simulink model "extra_blocks"  (R2023a)
settings: Solver=FixedStepDiscrete  StartTime=0.0  StopTime=inf  FixedStep=0.002  RelTol=1e-3  EnableMultiTasking=on
values from neighbouring files (symbols this model uses):
  a = 0    [simulate_hover.m]
  B = [0, 0, 0 ... (first row only)    [setup_lab_hover.m]    (also in simulate_hover.m = 0.042375883612; solveSyms3.m = evalin('base', 'B'))
  cycleGain = 0.2    [simulate_hover.m]    (also in temp.m = 1)
  Jp = 2*Jeq_prop    (= 0.0552224595625)    [setup_lab_hover.m]    (also in simulate_hover.m)
  Jr = 2*Jeq_prop    (= 0.0552224595625)    [setup_lab_hover.m]    (also in simulate_hover.m)
  Jy = 4*Jeq_prop    (= 0.110444919125)    [setup_lab_hover.m]    (also in simulate_hover.m)
  kd = 0.5    [simulate_hover.m]
  Kf = 0.1188    [setup_lab_hover.m]    (also in simulate_hover.m)
  Kt = 0.0036    [setup_lab_hover.m]    (also in simulate_hover.m)
  L = 7.75*0.0254    (= 0.19685)    [setup_lab_hover.m]    (also in simulate_hover.m = 0.1969)
  num1 = double(subs(u_1, {x1, x2, x3, x4, x5, x6, statey_der}, {v1, v2, v3, v4, v5, v6, v7}))    [solveSyms.m]
  num2 = double(subs(u_2, {x1, x2, x3, x4, x5, x6, u1}, {v1, v2, v3, v4, v5, v6, u1_num}))    [solveSyms.m]
  r = flexSize(no)    [phaseComp.m]    (also in simulate_hover.m = 0.5)
  skew = 2    [simulate_hover.m]
  u10_range = -199:100:401    [tempAdvanced.m]
  u1_range = -15:1:15    [tempAdvanced.m]
  V_bias = 12    [setup_lab_hover.m]    (also in simulate_hover.m)
  wcf = 2 * pi * 20    (= 125.663706144)    [setup_lab_hover.m]    (also in simulate_hover.m)
  x0 = x0(:)    [calc_jacob.m]    (also in setup_lab_hover.m = transpose(0.5*[pi/2, pi/6, pi/6, 0, 0, 0]))
  x5_range = -(29.5):10:(30.5)    [tempAdvanced.m]
  x6_range = -(29.5):10:(30.5)    [tempAdvanced.m]
  zetaf = 0.6    [setup_lab_hover.m]    (also in simulate_hover.m)
undefined symbols (not defined in the file or in its folder): Kp1_T, numBias, x1_range, x2_range
libraries: simulink_extras x3, quarc_library x2
settings Model: ExtModeTrigDuration=10000  Creator=kille  LastModifiedBy=Jacob
settings SolverCC: AlgebraicLoopSolver=TrustRegion  PositivePriorityOrder=on
settings DataIOCC: ReturnWorkspaceOutputs=off
settings OptimizationCC: LifeSpan=inf
settings DebuggingCC: UnconnectedInputMsg=warning  UnconnectedOutputMsg=warning  UnconnectedLineMsg=warning  ArithmeticOperatorsInVariantConditions=warning
settings ModelReferenceCC: EnableRefExpFcnMdlSchedulingChecks=on
settings SFSimCC: SimUseLocalCustomCode=off  CustomCodeUndefinedFunction=UseInterfaceOnly
settings RTWCC: Description=QUARC Win64 Target  SystemTargetFile=quarc_win64.tlc  TemplateMakefile=quarc_default_tmf  RTWUseLocalCustomCode=off
settings CodeAppCC: StateflowObjectComments=on
settings STFCustomTargetCC: TargetPreCompLibLocation=C:\PROGRA~3\QUARC\lib\2016a\win64\release  UseToolchainInfoCompliant=off  SystemTargetFile=quarc_win64.tlc
settings GRTTargetCC: TargetPreCompLibLocation=C:\PROGRA~3\QUARC\lib\2016a\win64\release  ParMdlRefBuildCompliant=off  CompOptLevelCompliant=off  CombineOutputUpdateFcns=off  MatFileLogging=off  CPPClassGenCompliant=off  GRTInterface=on  UseToolchainInfoCompliant=off  ExtMode=on  ExtModeMexFile=quarc_comm
settings ConfigComp: CovMetricSettings=dswe

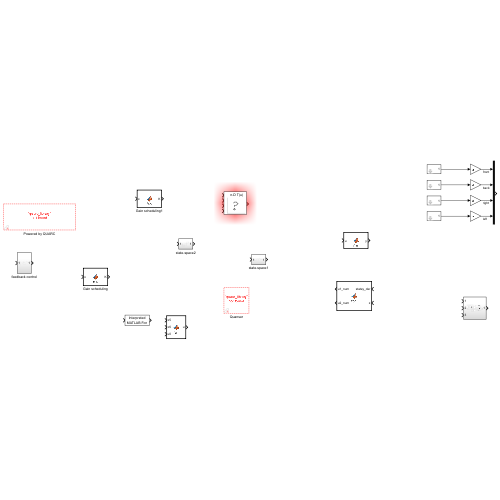
[thumbnail: Simulink's stored preview of the top-level diagram]
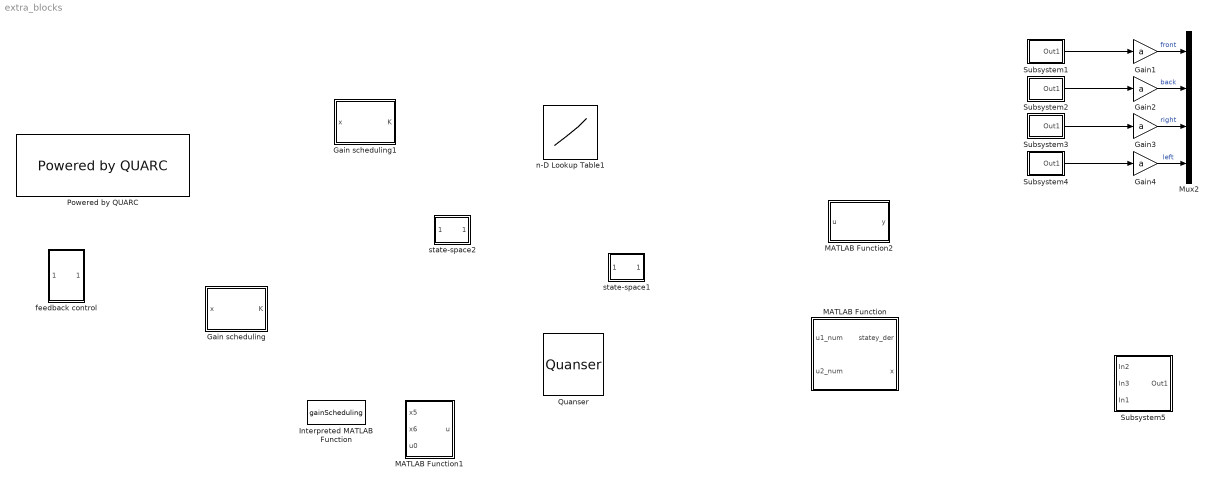
== system extra_blocks ==
  Gain scheduling : MATLAB Function  TreatAsAtomicUnit=on
  Gain scheduling1 : MATLAB Function  TreatAsAtomicUnit=on
  Gain{1..4} (4 alike) : Gain  Gain=a
  Interpreted MATLAB Function : MATLABFcn  MATLABFcn=gainScheduling  Output1D=off
  MATLAB Function : MATLAB Function  TreatAsAtomicUnit=on
  MATLAB Function1 : MATLAB Function  TreatAsAtomicUnit=on
  MATLAB Function2 : MATLAB Function  TreatAsAtomicUnit=on
  Mux2 : Mux
  Powered by QUARC : quarc_library/Logos/Powered by QUARC
  Quanser : quarc_library/Logos/Quanser
  Subsystem1 : Subsystem  mask{start_time=1, duration=1, amplitude=1}
      mask prompts: start_time "Start time"
  Subsystem2 : Subsystem  mask{start_time=6, duration=1, amplitude=1}
      mask prompts: start_time "Start time"
  Subsystem3 : Subsystem  mask{start_time=11, duration=1, amplitude=1}
      mask prompts: start_time "Start time"
  Subsystem4 : Subsystem  mask{start_time=16, duration=1, amplitude=1}
      mask prompts: start_time "Start time"
  Subsystem5 : Subsystem
  feedback control : Subsystem
  n-D Lookup Table1 : Lookup_n-D  NumberOfTableDimensions=4  BreakpointsForDimension1=x5_range  BreakpointsForDimension2=x6_range  BreakpointsForDimension3=u10_range  BreakpointsForDimension4=u20_range  Table=num2  InternalRulePriority=Speed  RndMeth=Simplest
      settings: InputPortMap=u0,u1,u2,u3
  state-space1 : Subsystem
  state-space2 : Subsystem
  wires:
  Subsystem2/1(Out1) -> Gain2/1
  Subsystem1/1(Out1) -> Gain1/1
  Subsystem3/1(Out1) -> Gain3/1
  Gain3/1 -> Mux2/3  "right"
  Gain4/1 -> Mux2/4  "left"
  Gain1/1 -> Mux2/1  "front"
  Gain2/1 -> Mux2/2  "back"
  Subsystem4/1(Out1) -> Gain4/1

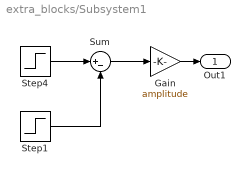
== system extra_blocks/Subsystem1 ==
  Gain : Gain  Gain=amplitude
  Step1 : Step  Time=start_time + duration  SampleTime=0
  Step4 : Step  Time=start_time  SampleTime=0
  Sum : Sum  Inputs=|+-
  Out1 : Outport
  wires:
  Gain/1 -> Out1/1
  Step1/1 -> Sum/2
  Step4/1 -> Sum/1
  Sum/1 -> Gain/1

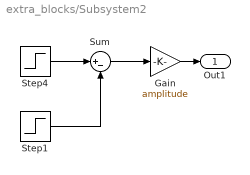
== system extra_blocks/Subsystem2 ==
  Gain : Gain  Gain=amplitude
  Step1 : Step  Time=start_time + duration  SampleTime=0
  Step4 : Step  Time=start_time  SampleTime=0
  Sum : Sum  Inputs=|+-
  Out1 : Outport
  wires:
  Gain/1 -> Out1/1
  Step1/1 -> Sum/2
  Step4/1 -> Sum/1
  Sum/1 -> Gain/1

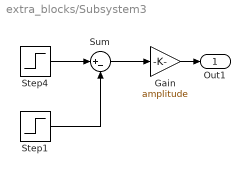
== system extra_blocks/Subsystem3 ==
  Gain : Gain  Gain=amplitude
  Step1 : Step  Time=start_time + duration  SampleTime=0
  Step4 : Step  Time=start_time  SampleTime=0
  Sum : Sum  Inputs=|+-
  Out1 : Outport
  wires:
  Gain/1 -> Out1/1
  Step1/1 -> Sum/2
  Step4/1 -> Sum/1
  Sum/1 -> Gain/1

== system extra_blocks/Subsystem4 ==
  Gain : Gain  Gain=amplitude
  Step1 : Step  Time=start_time + duration  SampleTime=0
  Step4 : Step  Time=start_time  SampleTime=0
  Sum : Sum  Inputs=|+-
  Out1 : Outport
  wires:
  Gain/1 -> Out1/1
  Step1/1 -> Sum/2
  Step4/1 -> Sum/1
  Sum/1 -> Gain/1

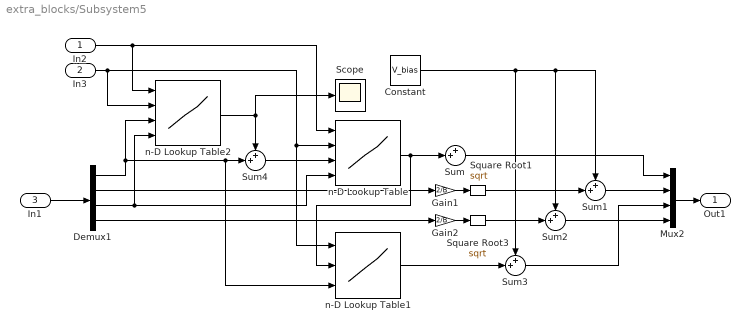
== system extra_blocks/Subsystem5 ==
  In2 : Inport
  In3 : Inport  Port=2
  In1 : Inport  Port=3
  Constant : Constant  Value=V_bias
  Demux1 : Demux
  Gain1 : Gain  Gain=2/B
  Gain2 : Gain  Gain=2/B
  Mux2 : Mux
  Scope : Scope
  Square Root1 : Sqrt
  Square Root3 : Sqrt
  Sum{,1..4} (5 alike) : Sum  Inputs=++|
  n-D Lookup Table : Lookup_n-D  NumberOfTableDimensions=4  BreakpointsForDimension1=x5_range  BreakpointsForDimension2=x6_range  BreakpointsForDimension3=u10_range  BreakpointsForDimension4=u20_range  Table=num1  InternalRulePriority=Speed  RndMeth=Simplest
      settings: InputPortMap=u0,u1,u2,u3
  n-D Lookup Table1 : Lookup_n-D  NumberOfTableDimensions=3  BreakpointsForDimension1=x6_range  BreakpointsForDimension2=u1_range  BreakpointsForDimension3=u10_range  BreakpointsForDimension4=u20_range  Table=num2  InternalRulePriority=Speed  RndMeth=Simplest
      settings: InputPortMap=u0,u1,u2
  n-D Lookup Table2 : Lookup_n-D  NumberOfTableDimensions=4  BreakpointsForDimension1=x5_range  BreakpointsForDimension2=x6_range  BreakpointsForDimension3=u10_range  BreakpointsForDimension4=u20_range  Table=numBias  InternalRulePriority=Speed  RndMeth=Simplest
      settings: InputPortMap=u0,u1,u2,u3
  Out1 : Outport
  wires:
  Demux1/2 -> Gain1/1
  In3/1 -> n-D Lookup Table2/2, n-D Lookup Table1/1, n-D Lookup Table/2
  n-D Lookup Table/1 -> Sum/2, n-D Lookup Table1/2
  Mux2/1 -> Out1/1
  Demux1/3 -> n-D Lookup Table2/4, n-D Lookup Table/4
  Gain2/1 -> Square Root3/1
  Demux1/4 -> Gain2/1
  In2/1 -> n-D Lookup Table2/1, n-D Lookup Table/1
  Gain1/1 -> Square Root1/1
  In1/1 -> Demux1/1
  Sum/1 -> Mux2/1
  Square Root3/1 -> Sum2/2
  Sum2/1 -> Mux2/4
  Square Root1/1 -> Sum1/2
  Sum1/1 -> Mux2/2
  Constant/1 -> Sum3/1, Sum2/1, Sum1/1
  Demux1/1 -> n-D Lookup Table1/3, Sum4/2, n-D Lookup Table2/3
  n-D Lookup Table2/1 -> Scope/1, Sum4/1
  n-D Lookup Table1/1 -> Sum3/2
  Sum3/1 -> Mux2/3
  Sum4/1 -> n-D Lookup Table/3

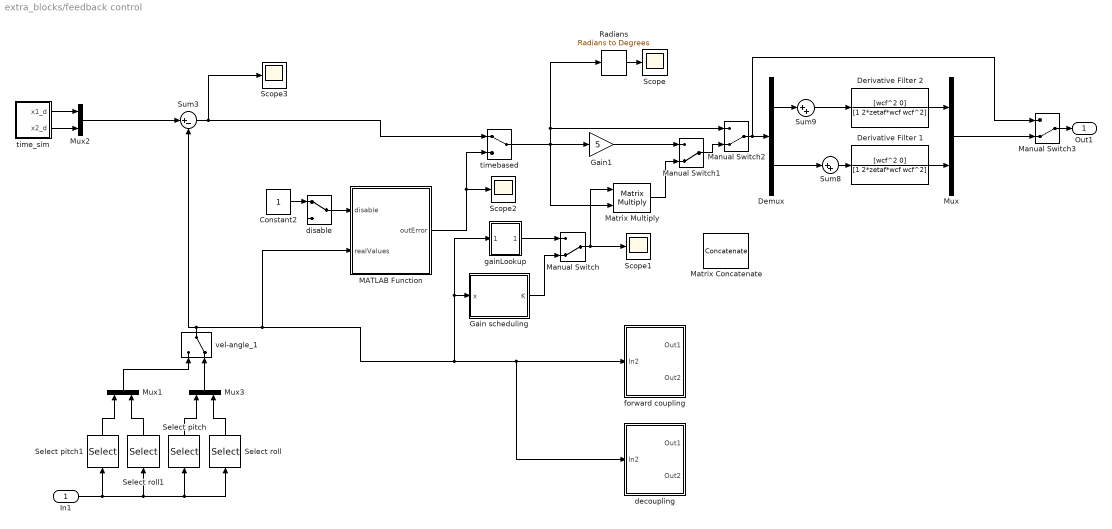
== system extra_blocks/feedback control ==
  In1 : Inport
  Constant2 : Constant
  Demux : Demux  Outputs=2
  Derivative Filter 1 : TransferFcn  Numerator=[wcf^2 0]  Denominator=[1 2*zetaf*wcf wcf^2]
  Derivative Filter 2 : TransferFcn  Numerator=[wcf^2 0]  Denominator=[1 2*zetaf*wcf wcf^2]
  Gain scheduling : MATLAB Function  TreatAsAtomicUnit=on
  Gain1 : Gain  Gain=5
  MATLAB Function : MATLAB Function  TreatAsAtomicUnit=on
  Manual Switch{,1..3} (4 alike) : ManualSwitch  CurrentSetting=0
  Matrix Concatenate : Concatenate  Mode=Multidimensional array  ConcatenateDimension=2
  Matrix Multiply : Product  Multiplication=Matrix(*)
  Mux{,1..3} (4 alike) : Mux  Inputs=2
  Radians : simulink_extras/Transformations/Radians to Degrees
  Scope{,1..3} (4 alike) : Scope
  Select pitch : Selector  InputPortWidth=6  IndexOptions=Index vector (dialog)  Indices=2  OutputSizes=1
  Select pitch1 : Selector  InputPortWidth=6  IndexOptions=Index vector (dialog)  Indices=5  OutputSizes=1
  Select roll : Selector  InputPortWidth=6  IndexOptions=Index vector (dialog)  Indices=3  OutputSizes=1
  Select roll1 : Selector  InputPortWidth=6  IndexOptions=Index vector (dialog)  Indices=6  OutputSizes=1
  Sum3 : Sum  Inputs=|+-
  Sum8 : Sum  Inputs=|++
  Sum9 : Sum  Inputs=|++
  decoupling : Subsystem
  disable : ManualSwitch
  forward coupling : Subsystem
  gainLookup : Subsystem
  time_sim : Subsystem
  timebased : ManualSwitch
  vel-angle_1 : ManualSwitch  CurrentSetting=0
  Out1 : Outport
  wires:
  In1/1 -> Select roll/1, Select pitch/1, Select roll1/1, Select pitch1/1
  Select pitch/1 -> Mux3/1
  time_sim/1(x1_d) -> Mux2/1
  time_sim/2(x2_d) -> Mux2/2
  Select roll/1 -> Mux3/2
  MATLAB Function/1(outError) -> Scope2/1, timebased/2
  Radians/1 -> Scope/1
  disable/1 -> MATLAB Function/1(disable)
  Constant2/1 -> disable/1
  Select roll1/1 -> Mux1/2
  Select pitch1/1 -> Mux1/1
  Mux1/1 -> vel-angle_1/1
  Mux3/1 -> vel-angle_1/2
  Mux2/1 -> Sum3/1
  Derivative Filter 2/1 -> Mux/1
  Derivative Filter 1/1 -> Mux/2
  Manual Switch2/1 -> Manual Switch3/1, Demux/1
  Manual Switch3/1 -> Out1/1
  Demux/2 -> Sum8/1
  Mux/1 -> Manual Switch3/2
  Sum8/1 -> Derivative Filter 1/1
  Sum9/1 -> Derivative Filter 2/1
  Demux/1 -> Sum9/1
  Sum3/1 -> Scope3/1, timebased/1
  Gain1/1 -> Manual Switch1/1
  timebased/1 -> Manual Switch2/1, Radians/1, Gain1/1, Matrix Multiply/2
  Manual Switch1/1 -> Manual Switch2/2
  Matrix Multiply/1 -> Manual Switch1/2
  vel-angle_1/1 -> Sum3/2, decoupling/1(In2), forward coupling/1(In2), gainLookup/1(In2), Gain scheduling/1(x), MATLAB Function/2(realValues)
  gainLookup/1(Out1) -> Manual Switch/1
  Manual Switch/1 -> Matrix Multiply/1, Scope1/1
  Gain scheduling/1(K) -> Manual Switch/2

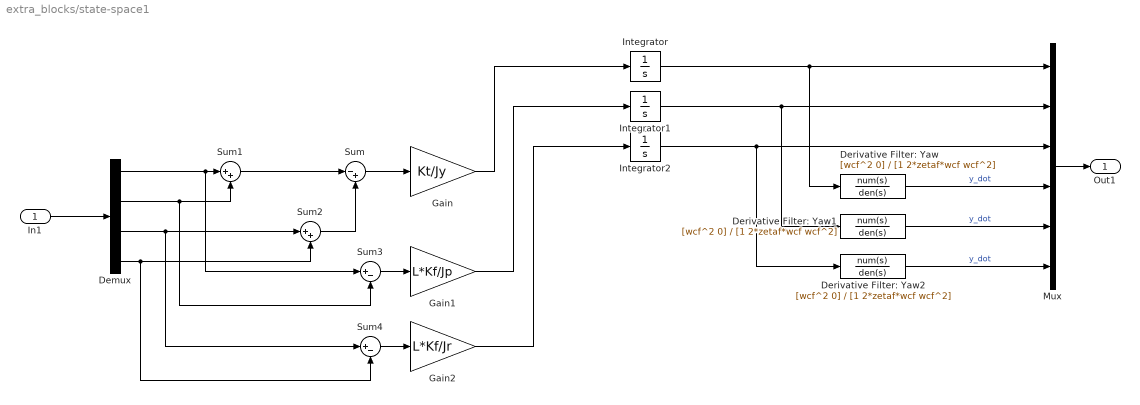
== system extra_blocks/state-space1 ==
  In1 : Inport
  Demux : Demux
  Derivative Filter: Yaw : TransferFcn  Numerator=[wcf^2 0]  Denominator=[1 2*zetaf*wcf wcf^2]
  Derivative Filter: Yaw1 : TransferFcn  Numerator=[wcf^2 0]  Denominator=[1 2*zetaf*wcf wcf^2]
  Derivative Filter: Yaw2 : TransferFcn  Numerator=[wcf^2 0]  Denominator=[1 2*zetaf*wcf wcf^2]
  Gain : Gain  Gain=Kt/Jy
  Gain1 : Gain  Gain=L*Kf/Jp
  Gain2 : Gain  Gain=L*Kf/Jr
  Integrator : Integrator  InitialCondition=x0(1)
  Integrator1 : Integrator  InitialCondition=x0(2)
  Integrator2 : Integrator  InitialCondition=x0(3)
  Mux : Mux  Inputs=6
  Sum : Sum  Inputs=|-+
  Sum1 : Sum  Inputs=|++
  Sum2 : Sum  Inputs=|++
  Sum3 : Sum  Inputs=|+-
  Sum4 : Sum  Inputs=|+-
  Out1 : Outport
  wires:
  In1/1 -> Demux/1
  Mux/1 -> Out1/1
  Sum/1 -> Gain/1
  Sum1/1 -> Sum/1
  Demux/1 -> Sum3/1, Sum1/1
  Demux/2 -> Sum1/2, Sum3/2
  Sum2/1 -> Sum/2
  Demux/3 -> Sum4/1, Sum2/1
  Demux/4 -> Sum4/2, Sum2/2
  Sum3/1 -> Gain1/1
  Sum4/1 -> Gain2/1
  Integrator/1 -> Derivative Filter: Yaw/1, Mux/1
  Integrator1/1 -> Derivative Filter: Yaw1/1, Mux/2
  Integrator2/1 -> Derivative Filter: Yaw2/1, Mux/3
  Gain2/1 -> Integrator2/1
  Gain1/1 -> Integrator1/1
  Gain/1 -> Integrator/1
  Derivative Filter: Yaw/1 -> Mux/4  "y_dot"
  Derivative Filter: Yaw1/1 -> Mux/5  "y_dot"
  Derivative Filter: Yaw2/1 -> Mux/6  "y_dot"

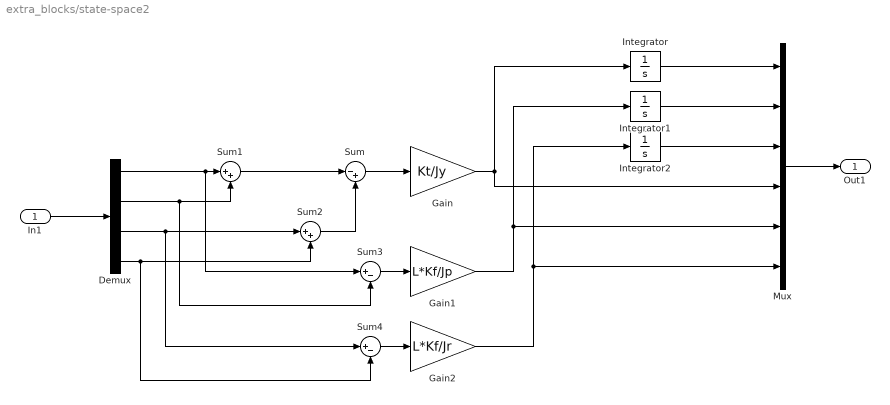
== system extra_blocks/state-space2 ==
  In1 : Inport
  Demux : Demux
  Gain : Gain  Gain=Kt/Jy
  Gain1 : Gain  Gain=L*Kf/Jp
  Gain2 : Gain  Gain=L*Kf/Jr
  Integrator : Integrator  InitialCondition=x0(1)
  Integrator1 : Integrator  InitialCondition=x0(2)
  Integrator2 : Integrator  InitialCondition=x0(3)
  Mux : Mux  Inputs=6
  Sum : Sum  Inputs=|-+
  Sum1 : Sum  Inputs=|++
  Sum2 : Sum  Inputs=|++
  Sum3 : Sum  Inputs=|+-
  Sum4 : Sum  Inputs=|+-
  Out1 : Outport
  wires:
  In1/1 -> Demux/1
  Mux/1 -> Out1/1
  Sum/1 -> Gain/1
  Sum1/1 -> Sum/1
  Demux/1 -> Sum3/1, Sum1/1
  Demux/2 -> Sum1/2, Sum3/2
  Sum2/1 -> Sum/2
  Demux/3 -> Sum4/1, Sum2/1
  Demux/4 -> Sum4/2, Sum2/2
  Sum3/1 -> Gain1/1
  Sum4/1 -> Gain2/1
  Integrator/1 -> Mux/1
  Integrator1/1 -> Mux/2
  Integrator2/1 -> Mux/3
  Gain/1 -> Integrator/1, Mux/4
  Gain1/1 -> Mux/5, Integrator1/1
  Gain2/1 -> Mux/6, Integrator2/1

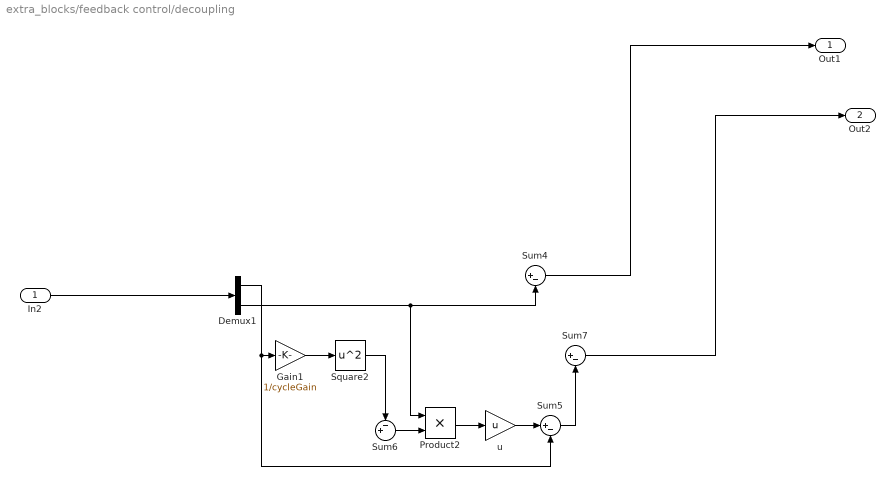
== system extra_blocks/feedback control/decoupling ==
  In2 : Inport
  Demux1 : Demux  Outputs=2
  Gain1 : Gain  Gain=1/cycleGain
  Product2 : Product
  Square2 : Math  Operator=square
  Sum4 : Sum  Inputs=|+-
  Sum5 : Sum  Inputs=|+-
  Sum6 : Sum  Inputs=-+|
  Sum7 : Sum  Inputs=|+-
  u : Gain  Gain=u
  Out1 : Outport
  Out2 : Outport  Port=2
  wires:
  Sum5/1 -> Sum7/2
  Sum7/1 -> Out2/1
  Square2/1 -> Sum6/1
  u/1 -> Sum5/1
  Demux1/1 -> Sum5/2, Gain1/1
  Product2/1 -> u/1
  Demux1/2 -> Product2/1, Sum4/2
  Sum6/1 -> Product2/2
  Gain1/1 -> Square2/1
  In2/1 -> Demux1/1
  Sum4/1 -> Out1/1

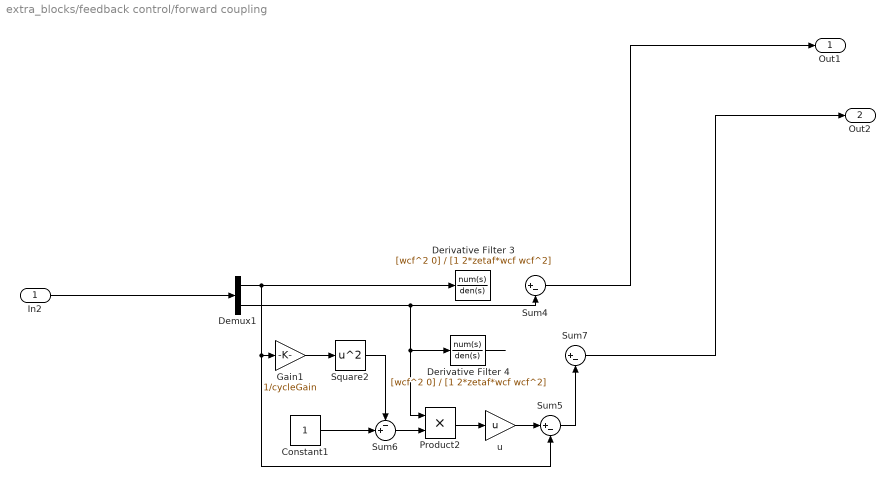
== system extra_blocks/feedback control/forward coupling ==
  In2 : Inport
  Constant1 : Constant
  Demux1 : Demux  Outputs=2
  Derivative Filter 3 : TransferFcn  Numerator=[wcf^2 0]  Denominator=[1 2*zetaf*wcf wcf^2]
  Derivative Filter 4 : TransferFcn  Numerator=[wcf^2 0]  Denominator=[1 2*zetaf*wcf wcf^2]
  Gain1 : Gain  Gain=1/cycleGain
  Product2 : Product
  Square2 : Math  Operator=square
  Sum4 : Sum  Inputs=|+-
  Sum5 : Sum  Inputs=|+-
  Sum6 : Sum  Inputs=-+|
  Sum7 : Sum  Inputs=|+-
  u : Gain  Gain=u
  Out1 : Outport
  Out2 : Outport  Port=2
  wires:
  Sum5/1 -> Sum7/2
  Sum7/1 -> Out2/1
  Square2/1 -> Sum6/1
  u/1 -> Sum5/1
  Demux1/1 -> Sum5/2, Gain1/1, Derivative Filter 3/1
  Product2/1 -> u/1
  Demux1/2 -> Product2/1, Derivative Filter 4/1, Sum4/2
  Sum6/1 -> Product2/2
  ? -> Sum7/1
  Constant1/1 -> Sum6/2
  Gain1/1 -> Square2/1
  In2/1 -> Demux1/1
  Sum4/1 -> Out1/1
  Derivative Filter 4/1 -> ?

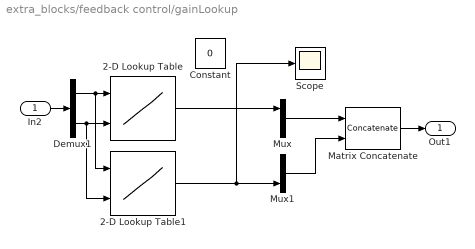
== system extra_blocks/feedback control/gainLookup ==
  In2 : Inport
  2-D Lookup Table : Lookup_n-D  BreakpointsForDimension1=x1_range  BreakpointsForDimension2=x2_range  Table=Kp1_T  InternalRulePriority=Speed  RndMeth=Simplest
      settings: InputPortMap=u0,u1
  2-D Lookup Table1 : Lookup_n-D  BreakpointsForDimension1=x1_range  BreakpointsForDimension2=x2_range  Table=Kp1_T  InternalRulePriority=Speed  RndMeth=Simplest
      settings: InputPortMap=u0,u1
  Constant : Constant  Value=0
  Demux1 : Demux  Outputs=2
  Matrix Concatenate : Concatenate  Mode=Multidimensional array  ConcatenateDimension=2
  Mux : Mux  Inputs=2
  Mux1 : Mux  Inputs=2
  Scope : Scope
  Out1 : Outport
  wires:
  In2/1 -> Demux1/1
  2-D Lookup Table/1 -> Mux/1
  2-D Lookup Table1/1 -> Scope/1, Mux1/2
  Mux/1 -> Matrix Concatenate/1
  Mux1/1 -> Matrix Concatenate/2
  Matrix Concatenate/1 -> Out1/1
  Demux1/1 -> 2-D Lookup Table1/1, 2-D Lookup Table/1
  Demux1/2 -> 2-D Lookup Table1/2, 2-D Lookup Table/2

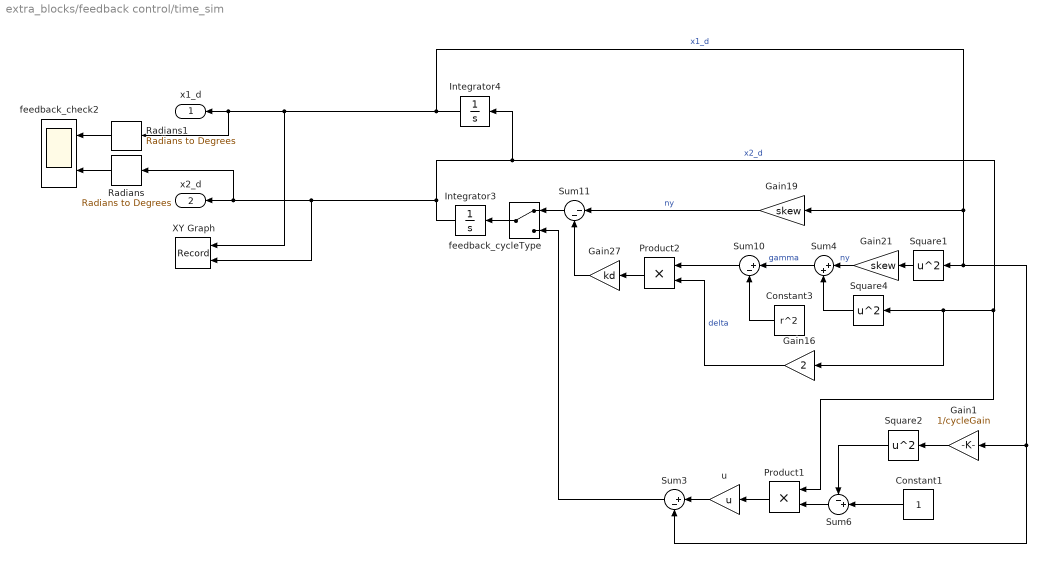
== system extra_blocks/feedback control/time_sim ==
  Constant1 : Constant
  Constant3 : Constant  Value=r^2
  Gain1 : Gain  Gain=1/cycleGain
  Gain16 : Gain  Gain=2
  Gain19 : Gain  Gain=skew
  Gain21 : Gain  Gain=skew
  Gain27 : Gain  Gain=kd
  Integrator3 : Integrator  InitialCondition=0.00010472
  Integrator4 : Integrator  InitialCondition=0.00010472
  Product1 : Product
  Product2 : Product
  Radians : simulink_extras/Transformations/Radians to Degrees
  Radians1 : simulink_extras/Transformations/Radians to Degrees
  Square1 : Math  Operator=square
  Square2 : Math  Operator=square
  Square4 : Math  Operator=square
  Sum10 : Sum  Inputs=|+-
  Sum11 : Sum  Inputs=|--
  Sum3 : Sum  Inputs=|+-
  Sum4 : Sum  Inputs=|++
  Sum6 : Sum  Inputs=-+|
  XY Graph : Record  FileSettingsInternal="{\"entries\":[{\"content\":{\"excelSettings\":{\"content\":{},\"type\":\"Streamout.ExcelSettings\"}},\"type\":\"Streamout.FileSettingStorage\",\"uuid\":\"\"}],\"packageUris\":[\"http:\\/\\/schema.mathworks.com\\/mf0\\/streamout_blocks\\/R2020a\"],\"version\":\"1.0\"}"  Layout=[1 1]  SignalsInternal="{\"entries\":[{\"content\":{\"signals\":[{\"content\":{\"blockPath\":[],\"dimensions\":[1],\"domain\":\"\",\"lineColor\":\"#a2142f\",\"plots\":[1],\"port\":1,\"signalID\":7111,\"signalName\":\"x1_d\"},\"type\":\"RecordBlkView.Signal\",\"uuid\":\"\"},{\"content\":{\"blockPath\":[],\"dimensions\":[1],\"domain\":\"\",\"lineColor\":\"#139fff\",\"plots\":[1],\"port\":2,\"signalID\":7114,\"signalName\":\"x2_d\"},\"type\":\"RecordBlkView.Signal\",\"uuid\":\"\"}]},\"type\":\"RecordBlkView.InputSignals\",\"uuid\":\"\"}],\"packageUris\":[\"http:\\/\\/schema.mathworks.com\\/mf0\\/streamout_blocks\\/R2020a\"],\"version\":\"1.0\"}"  VisualizationBindings="{\"xyplotplugin\":{\"info\":[{\"series\":[{\"bindingParametersList\":[{\"parameter\":\"X-Axis\",\"signalID\":7111,\"signalName\":\"x1_d\"},{\"parameter\":\"Y-Axis\",\"signalID\":7114,\"signalName\":\"x2_d\"}],\"seriesID\":48232}],\"subplotID\":1}]}}"  CompatibilityTag=XY
  feedback_check2 : Scope  NumInputPorts=2
  feedback_cycleType : ManualSwitch
  u : Gain  Gain=u
  x1_d : Outport
  x2_d : Outport  Port=2
  wires:
  Square1/1 -> Gain21/1
  Square4/1 -> Sum4/2
  Integrator4/1 -> Sum3/2, Gain1/1, Square1/1, Gain19/1, XY Graph/1, Radians1/1, x1_d/1  "x1_d"
  Gain27/1 -> Sum11/2
  Gain16/1 -> Product2/2  "delta"
  Gain19/1 -> Sum11/1  "ny"
  Integrator3/1 -> Product1/1, Gain16/1, Square4/1, Integrator4/1, XY Graph/2, Radians/1, x2_d/1  "x2_d"
  Sum10/1 -> Product2/1
  Constant3/1 -> Sum10/2
  Gain21/1 -> Sum4/1  "ny"
  Sum4/1 -> Sum10/1  "gamma"
  Product2/1 -> Gain27/1
  Radians1/1 -> feedback_check2/1
  Radians/1 -> feedback_check2/2
  Square2/1 -> Sum6/1
  Gain1/1 -> Square2/1
  u/1 -> Sum3/1
  Product1/1 -> u/1
  Sum6/1 -> Product1/2
  Constant1/1 -> Sum6/2
  feedback_cycleType/1 -> Integrator3/1
  Sum11/1 -> feedback_cycleType/1
  Sum3/1 -> feedback_cycleType/2

== matlab function extra_blocks/MATLAB Function1 ==
  data: x5 input; u output; x6 input; u0 input
function u = fcn(x5, x6, u0)
    %x1, x2, x3, x4, x5, x6 = x;
    coder.extrinsic('solveSyms2');
    u1 = 0;
    u2 = 0;
    [u1, u2] = solveSyms2(x5, x6, u0(1), u0(3));
    u = transpose([u1, 0, u2, 0]);
    %[u1, Vb, u2, Vl]
    Vl = 0;
    Vb = 0;
end

== matlab function extra_blocks/MATLAB Function ==
  data: statey_der input; x input; u1_num output; u2_num output
function [u1_num, u2_num] = fcn(statey_der, x)
    %x1, x2, x3, x4, x5, x6 = x;
    coder.extrinsic('solveSyms');
    u1_num = 0;
    u2_num = 0;
    [u1_num, u2_num] = solveSyms(x(1), x(2), x(3), x(4), x(5), x(6), statey_der);
end

== matlab function extra_blocks/MATLAB Function2 ==
  data: u input; y output
function y = fcn(u)

y = u;

V1^2 = max(-min)

== matlab function extra_blocks/Gain scheduling ==
  data: x input; K output
function K   = fcn(x)
    K = zeros(2);
    %Kr = zeros(2);
    %e = [0; 0];
    coder.extrinsic('gainScheduling');
    [K] = gainScheduling(x);
    %Kr = 1;
    %K = 50*eye(2);
    %K = [5, 0; 0, 50];
    
    %e = Kr*xv - K*x;
    %e = K*(xv - x);

== matlab function extra_blocks/feedback control/Gain scheduling ==
  data: x input; K output
function K   = fcn(x)
    K = zeros(2);
    %Kr = zeros(2);
    %e = [0; 0];
    coder.extrinsic('gainScheduling');
    [K] = gainScheduling(x);
    %Kr = 1;
    %K = 50*eye(2);
    %K = [5, 0; 0, 50];
    
    %e = Kr*xv - K*x;
    %e = K*(xv - x);

== matlab function extra_blocks/feedback control/MATLAB Function ==
  data: disable input; realValues input; outError output
function outError = approxLimitSimu(disable, realValues)
    outError = [0; 0];
    cyclePoint = [0; 0];
    %temp = load('paperCycle.mat');
    %cycleValues = temp.paperCycle;
    %for n = 1:2
    %    cycleN = cycleValues(:, n);
    %    realValueN = realValues(n);
    %    [closestValueError,idx]=min(abs(cycleN-realValueN));
    %    outError(n) = closestValueError;
    %end
    %disp(length(cycleValues))
    coder.extrinsic('approxLimit');
    coder.extrinsic('gainScheduling');
    if disable ~= 1
        cyclePoint = approxLimit(realValues);
        outError = cyclePoint-realValues;
        % K = [0, 0];
        % Km = zeros(2);
        % Kr = zeros(2);
        % K = gainScheduling(realValues);
        % Km = [K(1), 0; 0, K(2)];
        % outError = Km*(cyclePoint - realValues);
    end

== matlab function extra_blocks/Gain scheduling1 ==
  data: x input; K output
function K   = fcn(x)
    K = zeros(2, 4);
    %Kr = zeros(2);
    %e = [0; 0];
    coder.extrinsic('gainScheduling');
    [K] = gainScheduling(x);
    %Kr = 1;
    %K = 50*eye(2);
    %K = [5, 0; 0, 50];
    
    %e = Kr*xv - K*x;
    %e = K*(xv - x);
